simulink model "position_controller"  (R2021b)
settings: Solver=VariableStepAuto  StartTime=0.0  StopTime=10.0  RelTol=1e-3
settings Model: Creator=jcron  LastModifiedBy=jcron

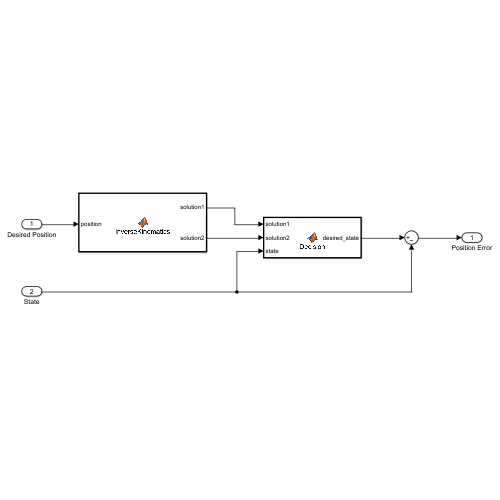
[thumbnail: Simulink's stored preview of the top-level diagram]
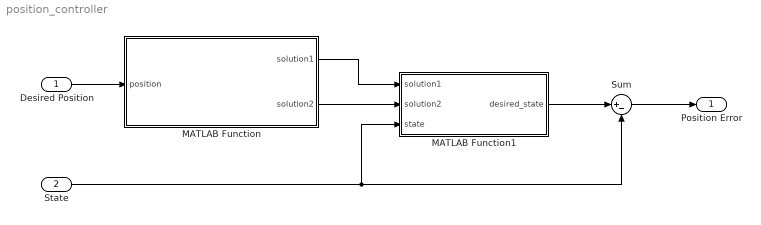
== system position_controller ==
  Desired Position : Inport
  State : Inport  Port=2
  MATLAB Function : MATLAB Function  TreatAsAtomicUnit=on
  MATLAB Function1 : MATLAB Function  TreatAsAtomicUnit=on
  Sum : Sum  Inputs=|+-
  Position Error : Outport
  wires:
  Desired Position/1 -> MATLAB Function/1(position)
  MATLAB Function/1(solution1) -> MATLAB Function1/1(solution1)
  MATLAB Function/2(solution2) -> MATLAB Function1/2(solution2)
  MATLAB Function1/1(desired_state) -> Sum/1
  Sum/1 -> Position Error/1
  State/1 -> Sum/2, MATLAB Function1/3(state)

== matlab function position_controller/MATLAB Function1 ==
  data: solution1 input; desired_state output; solution2 input; state input
function desired_state  = Decision(solution1, solution2, state)

desired_state = solution1;

== matlab function position_controller/MATLAB Function ==
  data: position input; solution1 output; solution2 output
function [solution1, solution2] = InverseKinematics(position)

end_eff_frame = expm(position(1) * skew3([1;0;0]));
end_eff_frame = end_eff_frame * expm(position(2) * skew3([0;1;0]));
end_eff_frame = end_eff_frame * expm(position(3) * skew3([0;0;1]));

all_solutions = inverseKinematics(end_eff_frame, pi / 2);

solution1 = all_solutions(1);
solution2 = all_solutions(2);
